simulink model "practica1_tp4_sim"  (R2025b)
settings: Solver=VariableStepAuto  StartTime=0.0  StopTime=320  MaxStep=T_p1/10  RelTol=1e-3
values from neighbouring files (symbols this model uses):
  A = [0   1         0 ... (first row only)    [TP4_practica1.m]    (also in TP4_practica4.m = [0 1 0)
  Ad = sys_d_c.A    [TP4_practica1.m]    (also in TP4_practica4.m)
  B = [0 ... (first row only)    [TP4_practica1.m]    (also in TP4_practica4.m)
  Bd = sys_d_c.B    [TP4_practica1.m]    (also in TP4_practica4.m)
  C = [1/N   0   0]    [TP4_practica1.m]    (also in TP4_practica4.m = [1 0 0])
  Cd = sys_d_c.C    [TP4_practica1.m]    (also in TP4_practica4.m)
  D = 0    [TP4_practica1.m]    (also in TP4_practica4.m)
  Ke1 = place(Ad',Cd',PolObsZ)'    [TP4_practica1.m]    (also in TP4_practica4.m)
  Ki1 = (Ki2_Ki1(4))'    [TP4_practica1.m]    (also in TP4_practica4.m)
  Ki2 = (Ki2_Ki1(1:3))'    [TP4_practica1.m]    (also in TP4_practica4.m)
  T_p1 = 1.109817844007972    (= 1.10981784401)    [TP4_practica1.m]

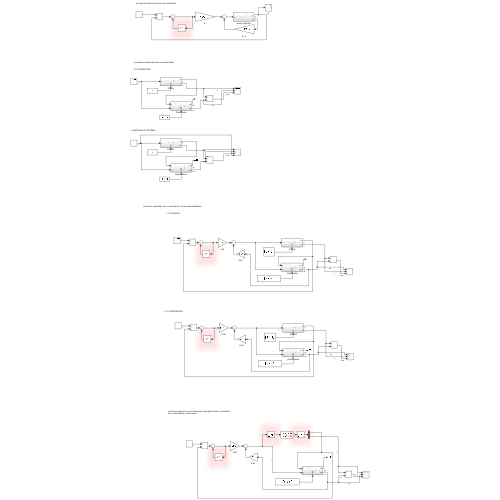
[thumbnail: Simulink's stored preview of the top-level diagram]
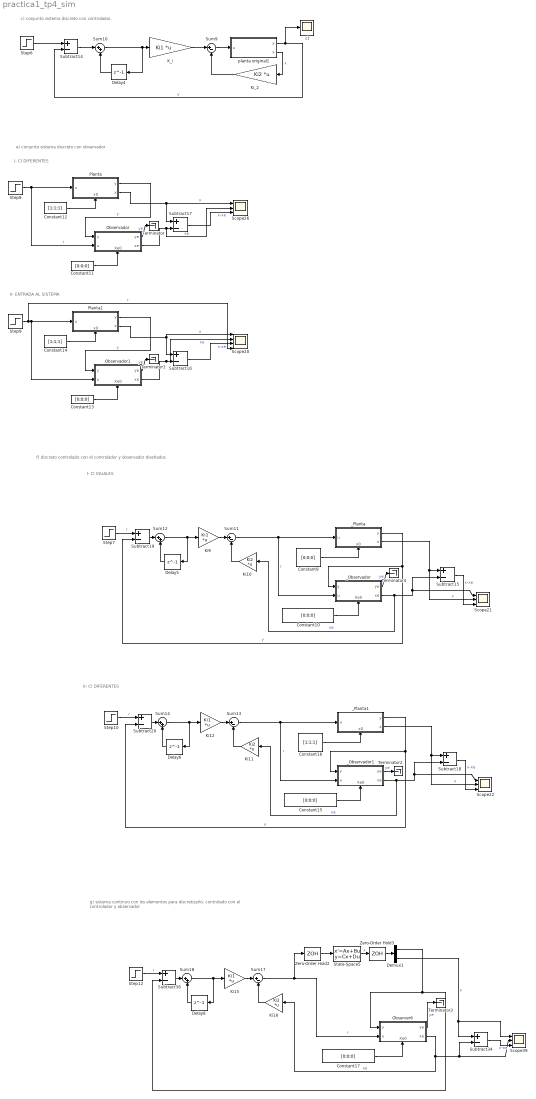
== system practica1_tp4_sim ==
  note: I- CI IGUALES
  note: I- CI DIFERENTES
  note: e) conjunto sistema discreto con observador
  note: II- ENTRADA AL SISTEMA
  note: f) discreto controlado con el controlador y observador diseñados
  note: II- CI DIFERENTES
  note: c) conjunto sistema discreto con controlador.
  note: g) sistema continuo con los elementos para discretizarlo, controlado
      | con el controlador y observador
  Constant{9..11,13,15,17} (6 alike) : Constant  Value=[0;0;0]
  Constant12 : Constant  Value=[1;1;1]
  Constant14 : Constant  Value=[1;1;1]
  Constant16 : Constant  Value=[1;1;1]
  Delay{4..6,8} (4 alike) : Delay  DelayLength=1  InitialCondition=0  SampleTime=T_p1
  Demux1 : Demux  Outputs=[1 3]
  K_i : Gain  Gain=Ki1  Multiplication=Matrix(K*u)
  Ki10 : Gain  Gain=Ki2  Multiplication=Matrix(K*u)
  Ki11 : Gain  Gain=Ki2  Multiplication=Matrix(K*u)
  Ki12 : Gain  Gain=Ki1  Multiplication=Matrix(K*u)
  Ki15 : Gain  Gain=Ki1  Multiplication=Matrix(K*u)
  Ki16 : Gain  Gain=Ki2  Multiplication=Matrix(K*u)
  Ki9 : Gain  Gain=Ki1  Multiplication=Matrix(K*u)
  Ki_2 : Gain  Gain=Ki2  Multiplication=Matrix(K*u)
  Observador : Subsystem
      settings: PortSchema="{\"entries\":[{\"content\":{\"sides\":[{\"content\":{\"connectorIds\":[\"In1\",\"In2\"]},\"type\":\"ConnectorPlacement.EquallySpacedRectSide\",\"uuid\":\"0206c41b-a718-4d7f-adb1-b10f19fec294\"},{\"content\":{\"connectorIds\":[\"Out1\",\"Out2\"],\"side\":\"RIGHT\"},\"type\":\"ConnectorPlacement.EquallySpacedRectSide\",\"uuid\":\"a2a8666a-9ec4-4b2c-aca8-860ba70d02d1\"},{\"content\":{\"connectorIds\":[],\"side\":\"TOP\"},\"type\":\"ConnectorPlacement.EquallySpacedRectSide\",\"uuid\":\"13e135fd-d3e9-457a-83a9-70769c6c120e\"},{\"content\":{\"connectorIds\":[\"In3\"],\"side\":\"BOTTOM\"},\"type\":\"ConnectorPlacement.EquallySpacedRectSide\",\"uuid\":\"a28a4721-1367-4666-b3df-1460e1b5a3ef\"}]},\"type\":\"ConnectorPlacement.EquallySpacedConnector\",\"uuid\":\"13d64113-8c44-41f3-9486-d2e1760fd679\"}],\"packageUris\":[\"http://schema.mathworks.com/mf0/Connector/19700101\"],\"version\":\"1.0\"}"
  Observador1 : Subsystem
      settings: PortSchema="{\"entries\":[{\"content\":{\"sides\":[{\"content\":{\"connectorIds\":[\"In1\",\"In2\"]},\"type\":\"ConnectorPlacement.EquallySpacedRectSide\",\"uuid\":\"0206c41b-a718-4d7f-adb1-b10f19fec294\"},{\"content\":{\"connectorIds\":[\"Out1\",\"Out2\"],\"side\":\"RIGHT\"},\"type\":\"ConnectorPlacement.EquallySpacedRectSide\",\"uuid\":\"a2a8666a-9ec4-4b2c-aca8-860ba70d02d1\"},{\"content\":{\"connectorIds\":[],\"side\":\"TOP\"},\"type\":\"ConnectorPlacement.EquallySpacedRectSide\",\"uuid\":\"13e135fd-d3e9-457a-83a9-70769c6c120e\"},{\"content\":{\"connectorIds\":[\"In3\"],\"side\":\"BOTTOM\"},\"type\":\"ConnectorPlacement.EquallySpacedRectSide\",\"uuid\":\"a28a4721-1367-4666-b3df-1460e1b5a3ef\"}]},\"type\":\"ConnectorPlacement.EquallySpacedConnector\",\"uuid\":\"13d64113-8c44-41f3-9486-d2e1760fd679\"}],\"packageUris\":[\"http://schema.mathworks.com/mf0/Connector/19700101\"],\"version\":\"1.0\"}"
  Observer6 : Subsystem
      settings: PortSchema="{\"entries\":[{\"content\":{\"sides\":[{\"content\":{\"connectorIds\":[\"In1\",\"In2\"]},\"type\":\"ConnectorPlacement.EquallySpacedRectSide\",\"uuid\":\"0206c41b-a718-4d7f-adb1-b10f19fec294\"},{\"content\":{\"connectorIds\":[\"Out1\",\"Out2\"],\"side\":\"RIGHT\"},\"type\":\"ConnectorPlacement.EquallySpacedRectSide\",\"uuid\":\"a2a8666a-9ec4-4b2c-aca8-860ba70d02d1\"},{\"content\":{\"connectorIds\":[],\"side\":\"TOP\"},\"type\":\"ConnectorPlacement.EquallySpacedRectSide\",\"uuid\":\"13e135fd-d3e9-457a-83a9-70769c6c120e\"},{\"content\":{\"connectorIds\":[\"In3\"],\"side\":\"BOTTOM\"},\"type\":\"ConnectorPlacement.EquallySpacedRectSide\",\"uuid\":\"a28a4721-1367-4666-b3df-1460e1b5a3ef\"}]},\"type\":\"ConnectorPlacement.EquallySpacedConnector\",\"uuid\":\"13d64113-8c44-41f3-9486-d2e1760fd679\"}],\"packageUris\":[\"http://schema.mathworks.com/mf0/Connector/19700101\"],\"version\":\"1.0\"}"
  Planta : Subsystem
      settings: PortSchema="{\"entries\":[{\"content\":{\"sides\":[{\"content\":{\"connectorIds\":[\"In1\"]},\"type\":\"ConnectorPlacement.EquallySpacedRectSide\",\"uuid\":\"f0fdeca5-2896-49f6-a4ba-0e1b68399016\"},{\"content\":{\"connectorIds\":[\"Out1\",\"Out2\"],\"side\":\"RIGHT\"},\"type\":\"ConnectorPlacement.EquallySpacedRectSide\",\"uuid\":\"8dec0bab-efad-4157-8acb-3883ca93220c\"},{\"content\":{\"side\":\"TOP\"},\"type\":\"ConnectorPlacement.EquallySpacedRectSide\",\"uuid\":\"dbbadfee-806e-4532-8aa9-9a5fb0f1d6b4\"},{\"content\":{\"connectorIds\":[\"In2\"],\"side\":\"BOTTOM\"},\"type\":\"ConnectorPlacement.EquallySpacedRectSide\",\"uuid\":\"88261f77-c9ac-43cd-91a6-42683e6f4e9c\"}]},\"type\":\"ConnectorPlacement.EquallySpacedConnector\",\"uuid\":\"deef2830-ef54-435a-a004-823eaca40138\"}],\"packageUris\":[\"http://schema.mathworks.com/mf0/Connector/R2020b\"],\"version\":\"1.0\"}"
  Planta1 : Subsystem
      settings: PortSchema="{\"entries\":[{\"content\":{\"sides\":[{\"content\":{\"connectorIds\":[\"In1\"]},\"type\":\"ConnectorPlacement.EquallySpacedRectSide\",\"uuid\":\"f0fdeca5-2896-49f6-a4ba-0e1b68399016\"},{\"content\":{\"connectorIds\":[\"Out1\",\"Out2\"],\"side\":\"RIGHT\"},\"type\":\"ConnectorPlacement.EquallySpacedRectSide\",\"uuid\":\"8dec0bab-efad-4157-8acb-3883ca93220c\"},{\"content\":{\"side\":\"TOP\"},\"type\":\"ConnectorPlacement.EquallySpacedRectSide\",\"uuid\":\"dbbadfee-806e-4532-8aa9-9a5fb0f1d6b4\"},{\"content\":{\"connectorIds\":[\"In2\"],\"side\":\"BOTTOM\"},\"type\":\"ConnectorPlacement.EquallySpacedRectSide\",\"uuid\":\"88261f77-c9ac-43cd-91a6-42683e6f4e9c\"}]},\"type\":\"ConnectorPlacement.EquallySpacedConnector\",\"uuid\":\"deef2830-ef54-435a-a004-823eaca40138\"}],\"packageUris\":[\"http://schema.mathworks.com/mf0/Connector/R2020b\"],\"version\":\"1.0\"}"
  Scope20 : Scope  NumInputPorts=4
      settings: ActiveDisplayYMinimum=-15.699510149714827  ActiveDisplayYMaximum=2.8555011277460913  DataLoggingVariableName=ScopeData22
  Scope{21..22,26,39} (4 alike) : Scope  NumInputPorts=3
      Scope21 settings: ActiveDisplayYMinimum=-1  ActiveDisplayYMaximum=1  DataLoggingVariableName=ScopeData24
      Scope22 settings: ActiveDisplayYMinimum=-1.7182016901748052  ActiveDisplayYMaximum=15.463815211560863  DataLoggingVariableName=ScopeData25
      Scope26 settings: ActiveDisplayYMinimum=-1.7182016901734991  ActiveDisplayYMaximum=15.463815211560718  DataLoggingVariableName=ScopeData29
      Scope39 settings: ActiveDisplayYMinimum=-2.7076623378974318E-6  ActiveDisplayYMaximum=6.2023665847732445E-7  DataLoggingVariableName=ScopeData42
  State-Space5 : StateSpace  A=A  B=B  C=[C;eye(3)]  D=[D;zeros(3,1)]  InitialCondition=0
  Step{6..7,10,12} (4 alike) : Step  Time=0  SampleTime=0
  Step8 : Step  Time=0  After=0  SampleTime=0
  Step9 : Step  Time=25  SampleTime=0
  Subtract{14..20,34,36} (9 alike) : Sum  Inputs=+-
  Sum{10,12,14,18} (4 alike) : Sum  Inputs=|++
  Sum{9,11,13,17} (4 alike) : Sum  Inputs=|+-
  Terminator{,1..4} (5 alike) : Terminator
  Zero-Order Hold2 : ZeroOrderHold  SampleTime=T_p1
  Zero-Order Hold3 : ZeroOrderHold  SampleTime=T_p1
  _Observador : Subsystem
      settings: PortSchema="{\"entries\":[{\"content\":{\"sides\":[{\"content\":{\"connectorIds\":[\"In1\",\"In2\"]},\"type\":\"ConnectorPlacement.EquallySpacedRectSide\",\"uuid\":\"0206c41b-a718-4d7f-adb1-b10f19fec294\"},{\"content\":{\"connectorIds\":[\"Out1\",\"Out2\"],\"side\":\"RIGHT\"},\"type\":\"ConnectorPlacement.EquallySpacedRectSide\",\"uuid\":\"a2a8666a-9ec4-4b2c-aca8-860ba70d02d1\"},{\"content\":{\"connectorIds\":[],\"side\":\"TOP\"},\"type\":\"ConnectorPlacement.EquallySpacedRectSide\",\"uuid\":\"13e135fd-d3e9-457a-83a9-70769c6c120e\"},{\"content\":{\"connectorIds\":[\"In3\"],\"side\":\"BOTTOM\"},\"type\":\"ConnectorPlacement.EquallySpacedRectSide\",\"uuid\":\"a28a4721-1367-4666-b3df-1460e1b5a3ef\"}]},\"type\":\"ConnectorPlacement.EquallySpacedConnector\",\"uuid\":\"13d64113-8c44-41f3-9486-d2e1760fd679\"}],\"packageUris\":[\"http://schema.mathworks.com/mf0/Connector/19700101\"],\"version\":\"1.0\"}"
  _Observador1 : Subsystem
      settings: PortSchema="{\"entries\":[{\"content\":{\"sides\":[{\"content\":{\"connectorIds\":[\"In1\",\"In2\"]},\"type\":\"ConnectorPlacement.EquallySpacedRectSide\",\"uuid\":\"0206c41b-a718-4d7f-adb1-b10f19fec294\"},{\"content\":{\"connectorIds\":[\"Out1\",\"Out2\"],\"side\":\"RIGHT\"},\"type\":\"ConnectorPlacement.EquallySpacedRectSide\",\"uuid\":\"a2a8666a-9ec4-4b2c-aca8-860ba70d02d1\"},{\"content\":{\"connectorIds\":[],\"side\":\"TOP\"},\"type\":\"ConnectorPlacement.EquallySpacedRectSide\",\"uuid\":\"13e135fd-d3e9-457a-83a9-70769c6c120e\"},{\"content\":{\"connectorIds\":[\"In3\"],\"side\":\"BOTTOM\"},\"type\":\"ConnectorPlacement.EquallySpacedRectSide\",\"uuid\":\"a28a4721-1367-4666-b3df-1460e1b5a3ef\"}]},\"type\":\"ConnectorPlacement.EquallySpacedConnector\",\"uuid\":\"13d64113-8c44-41f3-9486-d2e1760fd679\"}],\"packageUris\":[\"http://schema.mathworks.com/mf0/Connector/19700101\"],\"version\":\"1.0\"}"
  _Planta : Subsystem
      settings: PortSchema="{\"entries\":[{\"content\":{\"sides\":[{\"content\":{\"connectorIds\":[\"In1\"]},\"type\":\"ConnectorPlacement.EquallySpacedRectSide\",\"uuid\":\"f0fdeca5-2896-49f6-a4ba-0e1b68399016\"},{\"content\":{\"connectorIds\":[\"Out1\",\"Out2\"],\"side\":\"RIGHT\"},\"type\":\"ConnectorPlacement.EquallySpacedRectSide\",\"uuid\":\"8dec0bab-efad-4157-8acb-3883ca93220c\"},{\"content\":{\"side\":\"TOP\"},\"type\":\"ConnectorPlacement.EquallySpacedRectSide\",\"uuid\":\"dbbadfee-806e-4532-8aa9-9a5fb0f1d6b4\"},{\"content\":{\"connectorIds\":[\"In2\"],\"side\":\"BOTTOM\"},\"type\":\"ConnectorPlacement.EquallySpacedRectSide\",\"uuid\":\"88261f77-c9ac-43cd-91a6-42683e6f4e9c\"}]},\"type\":\"ConnectorPlacement.EquallySpacedConnector\",\"uuid\":\"deef2830-ef54-435a-a004-823eaca40138\"}],\"packageUris\":[\"http://schema.mathworks.com/mf0/Connector/R2020b\"],\"version\":\"1.0\"}"
  _Planta1 : Subsystem
      settings: PortSchema="{\"entries\":[{\"content\":{\"sides\":[{\"content\":{\"connectorIds\":[\"In1\"]},\"type\":\"ConnectorPlacement.EquallySpacedRectSide\",\"uuid\":\"f0fdeca5-2896-49f6-a4ba-0e1b68399016\"},{\"content\":{\"connectorIds\":[\"Out1\",\"Out2\"],\"side\":\"RIGHT\"},\"type\":\"ConnectorPlacement.EquallySpacedRectSide\",\"uuid\":\"8dec0bab-efad-4157-8acb-3883ca93220c\"},{\"content\":{\"side\":\"TOP\"},\"type\":\"ConnectorPlacement.EquallySpacedRectSide\",\"uuid\":\"dbbadfee-806e-4532-8aa9-9a5fb0f1d6b4\"},{\"content\":{\"connectorIds\":[\"In2\"],\"side\":\"BOTTOM\"},\"type\":\"ConnectorPlacement.EquallySpacedRectSide\",\"uuid\":\"88261f77-c9ac-43cd-91a6-42683e6f4e9c\"}]},\"type\":\"ConnectorPlacement.EquallySpacedConnector\",\"uuid\":\"deef2830-ef54-435a-a004-823eaca40138\"}],\"packageUris\":[\"http://schema.mathworks.com/mf0/Connector/R2020b\"],\"version\":\"1.0\"}"
  c) : Scope
      settings: ActiveDisplayYMinimum=-0.13745459748513414  ActiveDisplayYMaximum=1.2370913773662076  DataLoggingVariableName=ScopeData23
  planta original1 : Subsystem
  wires:
  Subtract14/1 -> Sum10/1
  K_i/1 -> Sum9/1
  planta original1/1(y) -> c)/1, Subtract14/2  "y"
  planta original1/2(x) -> Ki_2/1  "x"
  Ki_2/1 -> Sum9/2
  Delay4/1 -> Sum10/2
  Step6/1 -> Subtract14/1
  Sum9/1 -> planta original1/1(u)
  Sum10/1 -> K_i/1, Delay4/1
  Planta/1(y) -> Observador/1(y)  "y"
  Constant11/1 -> Observador/3(Xe0)
  Planta/2(x) -> Scope26/1, Subtract17/1  "x"
  Step8/1 -> Planta/1(u), Observador/2(u)  "r"
  Observador/2(xe) -> Subtract17/2, Scope26/2  "xe"
  Subtract17/1 -> Scope26/3  "x-xe"
  Constant12/1 -> Planta/2(x0)
  Observador/1(ye) -> Terminator/1  "ye"
  Sum12/1 -> Ki9/1, Delay5/1
  Subtract19/1 -> Sum12/1
  Constant10/1 -> _Observador/3(Xe0)
  Delay5/1 -> Sum12/2
  Subtract15/1 -> Scope21/3  "x-xe"
  Sum11/1 -> _Planta/1(u), _Observador/2(u)  "r"
  Step7/1 -> Subtract19/1  "r"
  Constant9/1 -> _Planta/2(x0)
  _Planta/2(x) -> Scope21/2, Subtract15/1  "x"
  _Observador/2(xe) -> Scope21/1, Subtract15/2, Ki10/1  "xe"
  _Planta/1(y) -> Subtract19/2, _Observador/1(y)  "y"
  Ki9/1 -> Sum11/1
  Ki10/1 -> Sum11/2
  Observador1/2(xe) -> Subtract16/2, Scope20/2  "xe"
  Constant13/1 -> Observador1/3(Xe0)
  Constant14/1 -> Planta1/2(x0)
  Planta1/2(x) -> Scope20/1, Subtract16/1  "x"
  Step9/1 -> Planta1/1(u), Observador1/2(u), Scope20/4  "r"
  Planta1/1(y) -> Observador1/1(y)  "y"
  Subtract16/1 -> Scope20/3  "x-xe"
  Observador1/1(ye) -> Terminator1/1  "ye"
  Ki12/1 -> Sum13/1
  _Planta1/2(x) -> Scope22/2, Subtract18/1  "x"
  Constant15/1 -> _Observador1/3(Xe0)
  Step10/1 -> Subtract20/1  "r"
  Subtract18/1 -> Scope22/3  "x-xe"
  Sum14/1 -> Ki12/1, Delay6/1
  Constant16/1 -> _Planta1/2(x0)
  _Planta1/1(y) -> Subtract20/2, _Observador1/1(y)  "y"
  Ki11/1 -> Sum13/2
  Subtract20/1 -> Sum14/1
  Delay6/1 -> Sum14/2
  _Observador1/2(xe) -> Scope22/1, Subtract18/2, Ki11/1  "xe"
  Sum13/1 -> _Planta1/1(u), _Observador1/2(u)  "r"
  Sum17/1 -> Zero-Order Hold2/1, Observer6/2(u)  "r"
  Step12/1 -> Subtract36/1  "r"
  Subtract36/1 -> Sum18/1
  Observer6/2(xe) -> Scope39/2, Subtract34/2, Ki16/1  "xe"
  Zero-Order Hold2/1 -> State-Space5/1
  Sum18/1 -> Ki15/1, Delay8/1
  Delay8/1 -> Sum18/2
  Ki16/1 -> Sum17/2
  Constant17/1 -> Observer6/3(Xe0)
  Ki15/1 -> Sum17/1
  _Observador1/1(ye) -> Terminator2/1  "ye"
  Subtract34/1 -> Scope39/3  "x-xe"
  State-Space5/1 -> Zero-Order Hold3/1  "x"
  Demux1/1 -> Observer6/1(y), Subtract36/2
  Observer6/1(ye) -> Terminator3/1  "ye"
  Zero-Order Hold3/1 -> Demux1/1
  Demux1/2 -> Scope39/1, Subtract34/1  "x"
  _Observador/1(ye) -> Terminator4/1  "ye"

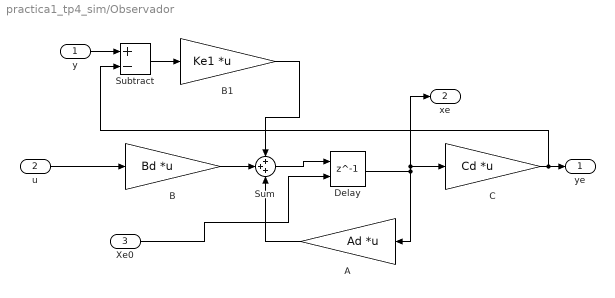
== system practica1_tp4_sim/Observador ==
  y : Inport
  u : Inport  Port=2
  Xe0 : Inport  Port=3
  A : Gain  Gain=Ad  Multiplication=Matrix(K*u)
  B : Gain  Gain=Bd  Multiplication=Matrix(K*u)
  B1 : Gain  Gain=Ke1  Multiplication=Matrix(K*u)
  C : Gain  Gain=Cd  Multiplication=Matrix(K*u)
  Delay : Delay  DelayLength=1  InitialConditionSource=Input port  InitialCondition=0  SampleTime=T_p1
      settings: InputPortMap=u0,p4
  Subtract : Sum  Inputs=+-
  Sum : Sum  Inputs=+++
  ye : Outport
  xe : Outport  Port=2
  wires:
  A/1 -> Sum/3
  Delay/1 -> xe/1, C/1, A/1
  B/1 -> Sum/2
  Sum/1 -> Delay/1
  u/1 -> B/1
  C/1 -> Subtract/2, ye/1
  B1/1 -> Sum/1
  Xe0/1 -> Delay/2
  y/1 -> Subtract/1
  Subtract/1 -> B1/1

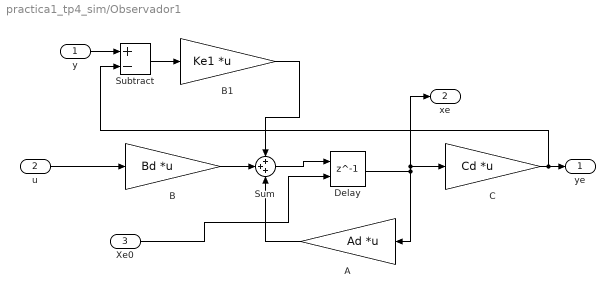
== system practica1_tp4_sim/Observador1 ==
  y : Inport
  u : Inport  Port=2
  Xe0 : Inport  Port=3
  A : Gain  Gain=Ad  Multiplication=Matrix(K*u)
  B : Gain  Gain=Bd  Multiplication=Matrix(K*u)
  B1 : Gain  Gain=Ke1  Multiplication=Matrix(K*u)
  C : Gain  Gain=Cd  Multiplication=Matrix(K*u)
  Delay : Delay  DelayLength=1  InitialConditionSource=Input port  InitialCondition=0  SampleTime=T_p1
      settings: InputPortMap=u0,p4
  Subtract : Sum  Inputs=+-
  Sum : Sum  Inputs=+++
  ye : Outport
  xe : Outport  Port=2
  wires:
  A/1 -> Sum/3
  Delay/1 -> xe/1, C/1, A/1
  B/1 -> Sum/2
  Sum/1 -> Delay/1
  u/1 -> B/1
  C/1 -> Subtract/2, ye/1
  B1/1 -> Sum/1
  Xe0/1 -> Delay/2
  y/1 -> Subtract/1
  Subtract/1 -> B1/1

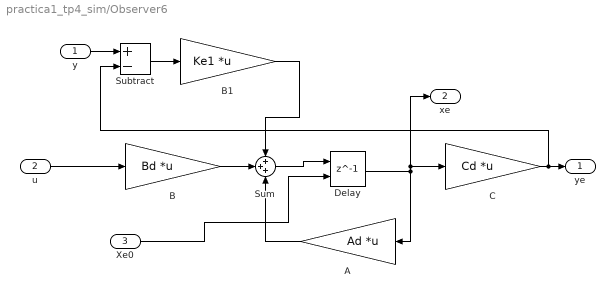
== system practica1_tp4_sim/Observer6 ==
  y : Inport
  u : Inport  Port=2
  Xe0 : Inport  Port=3
  A : Gain  Gain=Ad  Multiplication=Matrix(K*u)
  B : Gain  Gain=Bd  Multiplication=Matrix(K*u)
  B1 : Gain  Gain=Ke1  Multiplication=Matrix(K*u)
  C : Gain  Gain=Cd  Multiplication=Matrix(K*u)
  Delay : Delay  DelayLength=1  InitialConditionSource=Input port  InitialCondition=0  SampleTime=T_p1
      settings: InputPortMap=u0,p4
  Subtract : Sum  Inputs=+-
  Sum : Sum  Inputs=+++
  ye : Outport
  xe : Outport  Port=2
  wires:
  A/1 -> Sum/3
  Delay/1 -> xe/1, C/1, A/1
  B/1 -> Sum/2
  Sum/1 -> Delay/1
  u/1 -> B/1
  C/1 -> Subtract/2, ye/1
  B1/1 -> Sum/1
  Xe0/1 -> Delay/2
  y/1 -> Subtract/1
  Subtract/1 -> B1/1

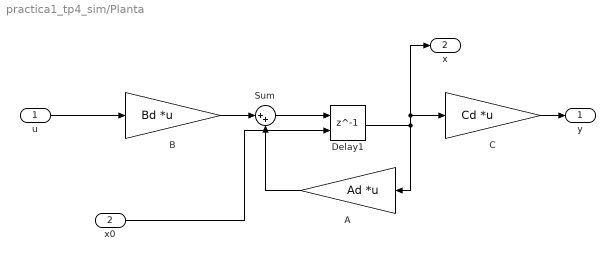
== system practica1_tp4_sim/Planta ==
  u : Inport
  x0 : Inport  Port=2
  A : Gain  Gain=Ad  Multiplication=Matrix(K*u)
  B : Gain  Gain=Bd  Multiplication=Matrix(K*u)
  C : Gain  Gain=Cd  Multiplication=Matrix(K*u)
  Delay1 : Delay  DelayLength=1  InitialConditionSource=Input port  InitialCondition=0  SampleTime=T_p1
      settings: InputPortMap=u0,p4
  Sum : Sum  Inputs=|++
  y : Outport
  x : Outport  Port=2
  wires:
  A/1 -> Sum/2
  Delay1/1 -> x/1, C/1, A/1
  B/1 -> Sum/1
  Sum/1 -> Delay1/1
  u/1 -> B/1
  C/1 -> y/1
  x0/1 -> Delay1/2

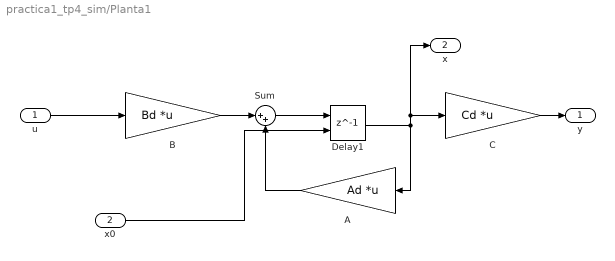
== system practica1_tp4_sim/Planta1 ==
  u : Inport
  x0 : Inport  Port=2
  A : Gain  Gain=Ad  Multiplication=Matrix(K*u)
  B : Gain  Gain=Bd  Multiplication=Matrix(K*u)
  C : Gain  Gain=Cd  Multiplication=Matrix(K*u)
  Delay1 : Delay  DelayLength=1  InitialConditionSource=Input port  InitialCondition=0  SampleTime=T_p1
      settings: InputPortMap=u0,p4
  Sum : Sum  Inputs=|++
  y : Outport
  x : Outport  Port=2
  wires:
  A/1 -> Sum/2
  Delay1/1 -> x/1, C/1, A/1
  B/1 -> Sum/1
  Sum/1 -> Delay1/1
  u/1 -> B/1
  C/1 -> y/1
  x0/1 -> Delay1/2

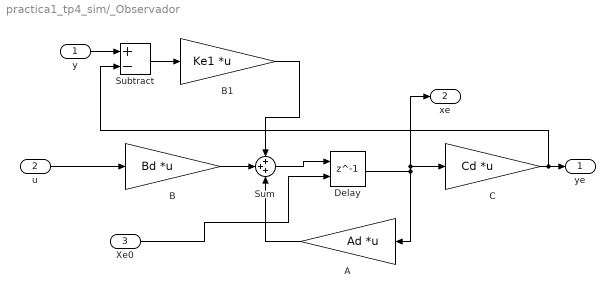
== system practica1_tp4_sim/_Observador ==
  y : Inport
  u : Inport  Port=2
  Xe0 : Inport  Port=3
  A : Gain  Gain=Ad  Multiplication=Matrix(K*u)
  B : Gain  Gain=Bd  Multiplication=Matrix(K*u)
  B1 : Gain  Gain=Ke1  Multiplication=Matrix(K*u)
  C : Gain  Gain=Cd  Multiplication=Matrix(K*u)
  Delay : Delay  DelayLength=1  InitialConditionSource=Input port  InitialCondition=0  SampleTime=T_p1
      settings: InputPortMap=u0,p4
  Subtract : Sum  Inputs=+-
  Sum : Sum  Inputs=+++
  ye : Outport
  xe : Outport  Port=2
  wires:
  A/1 -> Sum/3
  Delay/1 -> xe/1, C/1, A/1
  B/1 -> Sum/2
  Sum/1 -> Delay/1
  u/1 -> B/1
  C/1 -> Subtract/2, ye/1
  B1/1 -> Sum/1
  Xe0/1 -> Delay/2
  y/1 -> Subtract/1
  Subtract/1 -> B1/1

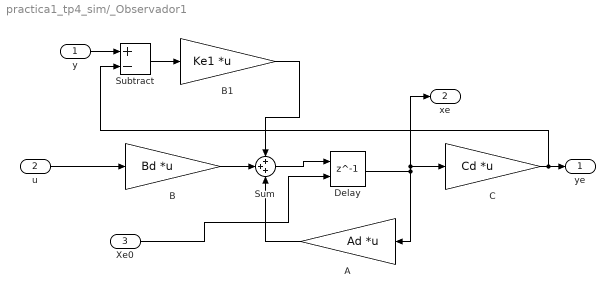
== system practica1_tp4_sim/_Observador1 ==
  y : Inport
  u : Inport  Port=2
  Xe0 : Inport  Port=3
  A : Gain  Gain=Ad  Multiplication=Matrix(K*u)
  B : Gain  Gain=Bd  Multiplication=Matrix(K*u)
  B1 : Gain  Gain=Ke1  Multiplication=Matrix(K*u)
  C : Gain  Gain=Cd  Multiplication=Matrix(K*u)
  Delay : Delay  DelayLength=1  InitialConditionSource=Input port  InitialCondition=0  SampleTime=T_p1
      settings: InputPortMap=u0,p4
  Subtract : Sum  Inputs=+-
  Sum : Sum  Inputs=+++
  ye : Outport
  xe : Outport  Port=2
  wires:
  A/1 -> Sum/3
  Delay/1 -> xe/1, C/1, A/1
  B/1 -> Sum/2
  Sum/1 -> Delay/1
  u/1 -> B/1
  C/1 -> Subtract/2, ye/1
  B1/1 -> Sum/1
  Xe0/1 -> Delay/2
  y/1 -> Subtract/1
  Subtract/1 -> B1/1

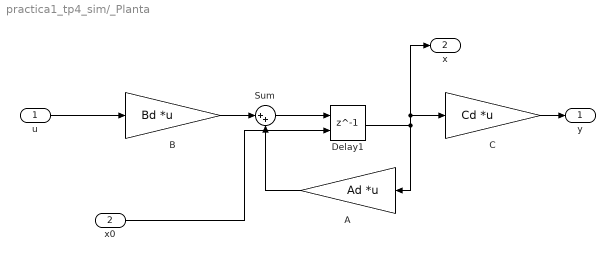
== system practica1_tp4_sim/_Planta ==
  u : Inport
  x0 : Inport  Port=2
  A : Gain  Gain=Ad  Multiplication=Matrix(K*u)
  B : Gain  Gain=Bd  Multiplication=Matrix(K*u)
  C : Gain  Gain=Cd  Multiplication=Matrix(K*u)
  Delay1 : Delay  DelayLength=1  InitialConditionSource=Input port  InitialCondition=0  SampleTime=T_p1
      settings: InputPortMap=u0,p4
  Sum : Sum  Inputs=|++
  y : Outport
  x : Outport  Port=2
  wires:
  A/1 -> Sum/2
  Delay1/1 -> x/1, C/1, A/1
  B/1 -> Sum/1
  Sum/1 -> Delay1/1
  u/1 -> B/1
  C/1 -> y/1
  x0/1 -> Delay1/2

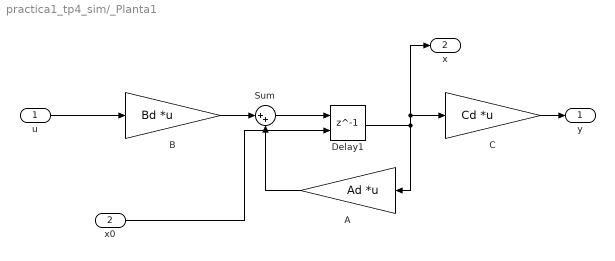
== system practica1_tp4_sim/_Planta1 ==
  u : Inport
  x0 : Inport  Port=2
  A : Gain  Gain=Ad  Multiplication=Matrix(K*u)
  B : Gain  Gain=Bd  Multiplication=Matrix(K*u)
  C : Gain  Gain=Cd  Multiplication=Matrix(K*u)
  Delay1 : Delay  DelayLength=1  InitialConditionSource=Input port  InitialCondition=0  SampleTime=T_p1
      settings: InputPortMap=u0,p4
  Sum : Sum  Inputs=|++
  y : Outport
  x : Outport  Port=2
  wires:
  A/1 -> Sum/2
  Delay1/1 -> x/1, C/1, A/1
  B/1 -> Sum/1
  Sum/1 -> Delay1/1
  u/1 -> B/1
  C/1 -> y/1
  x0/1 -> Delay1/2

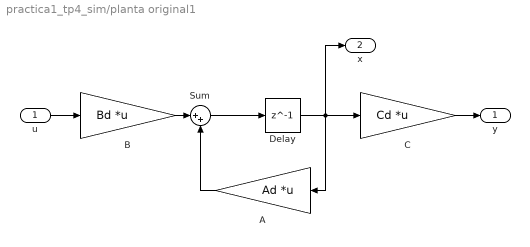
== system practica1_tp4_sim/planta original1 ==
  u : Inport
  A : Gain  Gain=Ad  Multiplication=Matrix(K*u)
  B : Gain  Gain=Bd  Multiplication=Matrix(K*u)
  C : Gain  Gain=Cd  Multiplication=Matrix(K*u)
  Delay : Delay  DelayLength=1  InitialCondition=0  SampleTime=T_p1
  Sum : Sum  Inputs=|++
  y : Outport
  x : Outport  Port=2
  wires:
  A/1 -> Sum/2
  Delay/1 -> x/1, C/1, A/1
  B/1 -> Sum/1
  Sum/1 -> Delay/1
  u/1 -> B/1
  C/1 -> y/1
